simulink model "State_Machine_Harness_Dashboard"  (R2019b)
settings: configuration reference "BMS_Sw_CodeGenConfig" (kept outside this file)
undefined symbols (not defined in the file): SRE
settings Model: DataDictionary=DD_State_Machine.sldd  Creator=falderis  LastModifiedBy=cpatel
settings ConfigSetRef: SourceName=BMS_Sw_CodeGenConfig

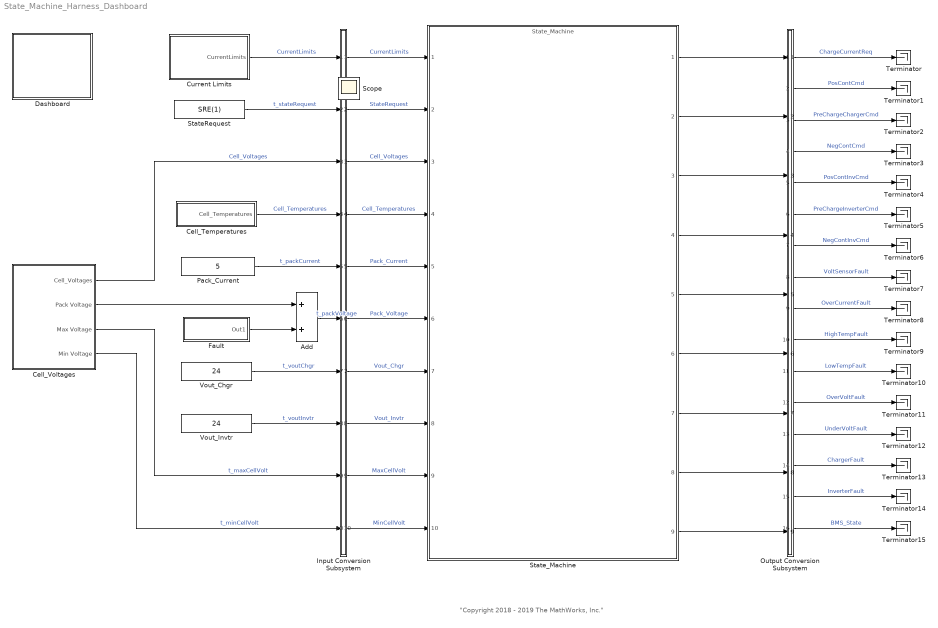
== system State_Machine_Harness_Dashboard ==
  note: "Copyright 2018 - 2019 The MathWorks, Inc."
  Add : Sum
  Cell_Temperatures : Subsystem
  Cell_Voltages : Subsystem
  Current Limits : Subsystem
  Dashboard : Subsystem
  Fault : Subsystem
  Input Conversion Subsystem : Subsystem  Tag=__SLT_ICS__  Description=|
      | Signal spec.
      | and routing
      settings: AttributesFormatString=%<Description>
  Output Conversion Subsystem : Subsystem  Tag=__SLT_OCS__  Description=|
      | Signal spec.
      | and routing
      settings: AttributesFormatString=%<Description>
  Pack_Current : Constant  Value=5  OutDataTypeStr=single  SampleTime=0.1
  StateRequest : Constant  Value=SRE(1)  OutDataTypeStr=Enum: SRE  SampleTime=0.1
  State_Machine : ModelReference  ModelNameDialog=State_Machine  SimulationMode=Normal  ModelReferenceVersion=1.640
  Terminator{,1..15} (16 alike) : Terminator
  Vout_Chgr : Constant  Value=24  OutDataTypeStr=single  SampleTime=0.1
  Vout_Invtr : Constant  Value=24  OutDataTypeStr=single  SampleTime=0.1
  Scope : Scope
  wires:
  Output Conversion Subsystem/1(Outport_1) -> Terminator/1  "ChargeCurrentReq"
  Output Conversion Subsystem/2(Outport_2) -> Terminator1/1  "PosContCmd"
  Output Conversion Subsystem/3(Outport_3) -> Terminator2/1  "PreChargeChargerCmd"
  Output Conversion Subsystem/4(Outport_4) -> Terminator3/1  "NegContCmd"
  Output Conversion Subsystem/5(Outport_5) -> Terminator4/1  "PosContInvCmd"
  Output Conversion Subsystem/6(Outport_6) -> Terminator5/1  "PreChargeInverterCmd"
  Output Conversion Subsystem/7(Outport_7) -> Terminator6/1  "NegContInvCmd"
  Output Conversion Subsystem/8(Outport_8) -> Terminator7/1  "VoltSensorFault"
  Output Conversion Subsystem/9(Outport_9) -> Terminator8/1  "OverCurrentFault"
  Output Conversion Subsystem/10(Outport_10) -> Terminator9/1  "HighTempFault"
  Output Conversion Subsystem/11(Outport_11) -> Terminator10/1  "LowTempFault"
  Output Conversion Subsystem/12(Outport_12) -> Terminator11/1  "OverVoltFault"
  Output Conversion Subsystem/13(Outport_13) -> Terminator12/1  "UnderVoltFault"
  Output Conversion Subsystem/14(Outport_14) -> Terminator13/1  "ChargerFault"
  Output Conversion Subsystem/15(Outport_15) -> Terminator14/1  "InverterFault"
  Output Conversion Subsystem/16(Outport_16) -> Terminator15/1  "BMS_State"
  Input Conversion Subsystem/1(Outport_1) -> State_Machine/1  "CurrentLimits"
  Input Conversion Subsystem/2(Outport_2) -> State_Machine/2  "StateRequest"
  Input Conversion Subsystem/3(Outport_3) -> State_Machine/3  "Cell_Voltages"
  Input Conversion Subsystem/4(Outport_4) -> State_Machine/4  "Cell_Temperatures"
  Input Conversion Subsystem/5(Outport_5) -> State_Machine/5  "Pack_Current"
  Input Conversion Subsystem/6(Outport_6) -> State_Machine/6  "Pack_Voltage"
  Input Conversion Subsystem/7(Outport_7) -> State_Machine/7  "Vout_Chgr"
  Input Conversion Subsystem/8(Outport_8) -> State_Machine/8  "Vout_Invtr"
  Input Conversion Subsystem/9(Outport_9) -> State_Machine/9  "MaxCellVolt"
  Input Conversion Subsystem/10(Outport_10) -> State_Machine/10  "MinCellVolt"
  State_Machine/1 -> Output Conversion Subsystem/1(Inport_1)
  State_Machine/2 -> Output Conversion Subsystem/2(Inport_2)
  State_Machine/3 -> Output Conversion Subsystem/3(Inport_3)
  State_Machine/4 -> Output Conversion Subsystem/4(Inport_4)
  State_Machine/5 -> Output Conversion Subsystem/5(Inport_5)
  State_Machine/6 -> Output Conversion Subsystem/6(Inport_6)
  State_Machine/7 -> Output Conversion Subsystem/7(Inport_7)
  State_Machine/8 -> Output Conversion Subsystem/8(Inport_8)
  State_Machine/9 -> Output Conversion Subsystem/9(Inport_9)
  Cell_Voltages/3(Max Voltage) -> Input Conversion Subsystem/9(Inport_9)  "t_maxCellVolt"
  Vout_Invtr/1 -> Input Conversion Subsystem/8(Inport_8)  "t_voutInvtr"
  Vout_Chgr/1 -> Input Conversion Subsystem/7(Inport_7)  "t_voutChgr"
  StateRequest/1 -> Input Conversion Subsystem/2(Inport_2)  "t_stateRequest"
  Cell_Voltages/4(Min Voltage) -> Input Conversion Subsystem/10(Inport_10)  "t_minCellVolt"
  Add/1 -> Input Conversion Subsystem/6(Inport_6)  "t_packVoltage"
  Current Limits/1(CurrentLimits) -> Input Conversion Subsystem/1(Inport_1)  "CurrentLimits"
  Cell_Temperatures/1(Cell_Temperatures) -> Input Conversion Subsystem/4(Inport_4)  "Cell_Temperatures"
  Cell_Voltages/1(Cell_Voltages) -> Input Conversion Subsystem/3(Inport_3)  "Cell_Voltages"
  Pack_Current/1 -> Input Conversion Subsystem/5(Inport_5)  "t_packCurrent"
  Cell_Voltages/2(Pack Voltage) -> Add/1
  Fault/1(Out1) -> Add/2

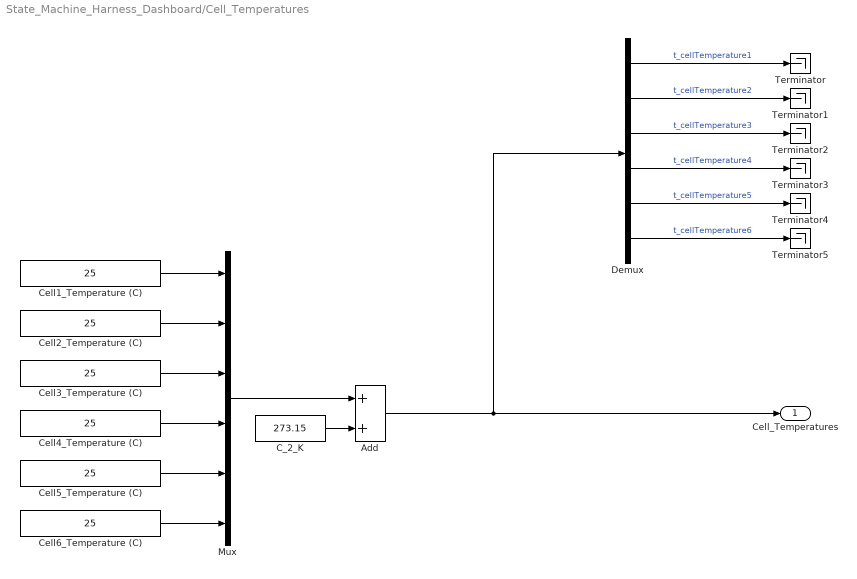
== system State_Machine_Harness_Dashboard/Cell_Temperatures ==
  Add : Sum
  C_2_K : Constant  Value=273.15  OutDataTypeStr=single  SampleTime=0.1
  Cell1_Temperature (C) : Constant  Value=25  OutDataTypeStr=single  SampleTime=0.1
  Cell2_Temperature (C) : Constant  Value=25  OutDataTypeStr=single  SampleTime=0.1
  Cell3_Temperature (C) : Constant  Value=25  OutDataTypeStr=single  SampleTime=0.1
  Cell4_Temperature (C) : Constant  Value=25  OutDataTypeStr=single  SampleTime=0.1
  Cell5_Temperature (C) : Constant  Value=25  OutDataTypeStr=single  SampleTime=0.1
  Cell6_Temperature (C) : Constant  Value=25  OutDataTypeStr=single  SampleTime=0.1
  Demux : Demux  Outputs=6
  Mux : Mux  Inputs=6
  Terminator{,1..5} (6 alike) : Terminator
  Cell_Temperatures : Outport  VectorParamsAs1DForOutWhenUnconnected=off
  wires:
  Add/1 -> Demux/1, Cell_Temperatures/1
  Cell3_Temperature (C)/1 -> Mux/3
  C_2_K/1 -> Add/2
  Cell2_Temperature (C)/1 -> Mux/2
  Cell4_Temperature (C)/1 -> Mux/4
  Cell5_Temperature (C)/1 -> Mux/5
  Mux/1 -> Add/1
  Cell6_Temperature (C)/1 -> Mux/6
  Cell1_Temperature (C)/1 -> Mux/1
  Demux/1 -> Terminator/1  "t_cellTemperature1"
  Demux/2 -> Terminator1/1  "t_cellTemperature2"
  Demux/3 -> Terminator2/1  "t_cellTemperature3"
  Demux/4 -> Terminator3/1  "t_cellTemperature4"
  Demux/5 -> Terminator4/1  "t_cellTemperature5"
  Demux/6 -> Terminator5/1  "t_cellTemperature6"

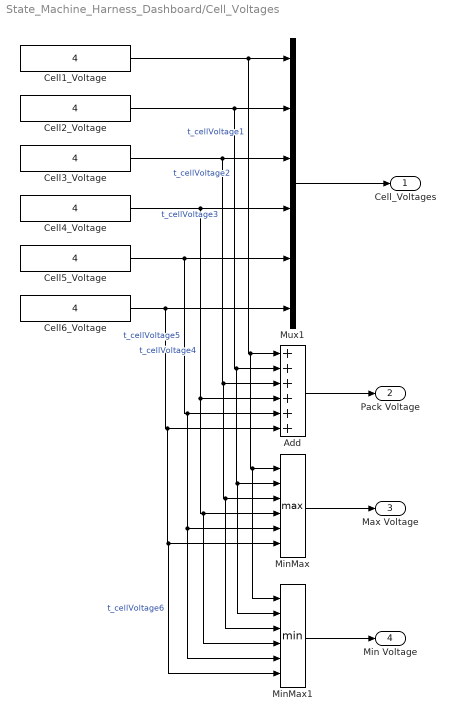
== system State_Machine_Harness_Dashboard/Cell_Voltages ==
  Add : Sum  Inputs=6
  Cell1_Voltage : Constant  Value=4  OutDataTypeStr=single  SampleTime=0.1
  Cell2_Voltage : Constant  Value=4  OutDataTypeStr=single  SampleTime=0.1
  Cell3_Voltage : Constant  Value=4  OutDataTypeStr=single  SampleTime=0.1
  Cell4_Voltage : Constant  Value=4  OutDataTypeStr=single  SampleTime=0.1
  Cell5_Voltage : Constant  Value=4  OutDataTypeStr=single  SampleTime=0.1
  Cell6_Voltage : Constant  Value=4  OutDataTypeStr=single  SampleTime=0.1
  MinMax : MinMax  Function=max  Inputs=6
  MinMax1 : MinMax  Inputs=6
  Mux1 : Mux  Inputs=6
  Cell_Voltages : Outport  VectorParamsAs1DForOutWhenUnconnected=off
  Pack Voltage : Outport  Port=2  VectorParamsAs1DForOutWhenUnconnected=off
  Max Voltage : Outport  Port=3  VectorParamsAs1DForOutWhenUnconnected=off
  Min Voltage : Outport  Port=4  VectorParamsAs1DForOutWhenUnconnected=off
  wires:
  Cell6_Voltage/1 -> MinMax1/6, MinMax/6, Add/6, Mux1/6  "t_cellVoltage6"
  Cell3_Voltage/1 -> MinMax1/3, MinMax/3, Add/3, Mux1/3  "t_cellVoltage3"
  Cell2_Voltage/1 -> MinMax1/2, MinMax/2, Add/2, Mux1/2  "t_cellVoltage2"
  Mux1/1 -> Cell_Voltages/1
  Cell1_Voltage/1 -> MinMax1/1, MinMax/1, Add/1, Mux1/1  "t_cellVoltage1"
  Cell5_Voltage/1 -> MinMax1/5, MinMax/5, Add/5, Mux1/5  "t_cellVoltage5"
  Cell4_Voltage/1 -> MinMax1/4, MinMax/4, Add/4, Mux1/4  "t_cellVoltage4"
  Add/1 -> Pack Voltage/1
  MinMax/1 -> Max Voltage/1
  MinMax1/1 -> Min Voltage/1

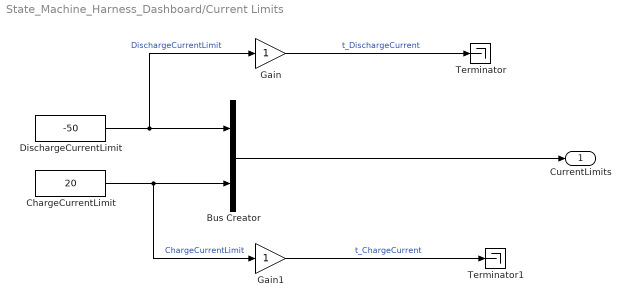
== system State_Machine_Harness_Dashboard/Current Limits ==
  Bus Creator : BusCreator  Inputs=2  OutDataTypeStr=Bus: CurrentLimits
  ChargeCurrentLimit : Constant  Value=20  OutDataTypeStr=single  SampleTime=0.1
  DischargeCurrentLimit : Constant  Value=-50  OutDataTypeStr=single  SampleTime=0.1
  Gain : Gain
  Gain1 : Gain
  Terminator : Terminator
  Terminator1 : Terminator
  CurrentLimits : Outport  VectorParamsAs1DForOutWhenUnconnected=off
  wires:
  Bus Creator/1 -> CurrentLimits/1
  DischargeCurrentLimit/1 -> Gain/1, Bus Creator/1  "DischargeCurrentLimit"
  ChargeCurrentLimit/1 -> Gain1/1, Bus Creator/2  "ChargeCurrentLimit"
  Gain/1 -> Terminator/1  "t_DischargeCurrent"
  Gain1/1 -> Terminator1/1  "t_ChargeCurrent"

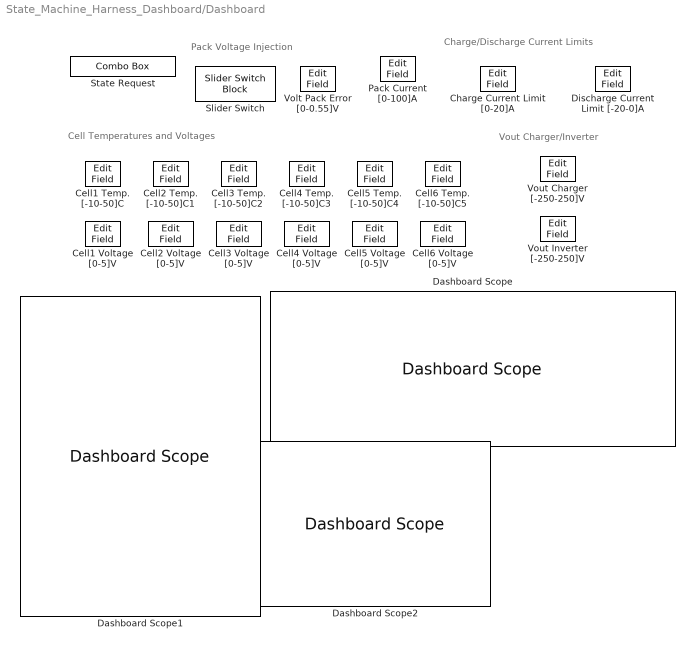
== system State_Machine_Harness_Dashboard/Dashboard ==
  note: Pack Voltage Injection
  note: Cell Temperatures and Voltages
  note: Vout Charger/Inverter
  note: Charge/Discharge Current Limits
  Cell1 Temp. [-10-50]C : EditField  LabelPosition=Hide  ShowInitialText=on  Alignment=Center
  Cell1 Voltage [0-5]V : EditField  LabelPosition=Hide  ShowInitialText=on  Alignment=Center
  Cell2 Temp. [-10-50]C1 : EditField  LabelPosition=Hide  ShowInitialText=on  Alignment=Center
  Cell2 Voltage [0-5]V : EditField  LabelPosition=Hide  ShowInitialText=on  Alignment=Center
  Cell3 Temp. [-10-50]C2 : EditField  LabelPosition=Hide  ShowInitialText=on  Alignment=Center
  Cell3 Voltage [0-5]V : EditField  LabelPosition=Hide  ShowInitialText=on  Alignment=Center
  Cell4 Temp. [-10-50]C3 : EditField  LabelPosition=Hide  ShowInitialText=on  Alignment=Center
  Cell4 Voltage [0-5]V : EditField  LabelPosition=Hide  ShowInitialText=on  Alignment=Center
  Cell5 Temp. [-10-50]C4 : EditField  LabelPosition=Hide  ShowInitialText=on  Alignment=Center
  Cell5 Voltage [0-5]V : EditField  LabelPosition=Hide  ShowInitialText=on  Alignment=Center
  Cell6 Temp. [-10-50]C5 : EditField  LabelPosition=Hide  ShowInitialText=on  Alignment=Center
  Cell6 Voltage [0-5]V : EditField  LabelPosition=Hide  ShowInitialText=on  Alignment=Center
  Charge Current Limit [0-20]A : EditField  LabelPosition=Hide  ShowInitialText=on  Alignment=Center
  Dashboard Scope : DashboardScope  TimeSpan=50  ScaleAtStop=off
  Dashboard Scope1 : DashboardScope  TimeSpan=50  Ymin=0  Ymax=1.2
  Dashboard Scope2 : DashboardScope  TimeSpan=50  Ymin=0  Ymax=35
  Discharge Current Limit [-20-0]A : EditField  LabelPosition=Hide  ShowInitialText=on  Alignment=Center
  Pack Current [0-100]A : EditField  LabelPosition=Hide  ShowInitialText=on  Alignment=Center
  Slider Switch : SliderSwitchBlock
      settings: Values={{'Off', 'On'}, [0 1]}
  State Request : ComboBox  LabelPosition=Hide  SelectedLabel=Charging
      settings: Values={{'Balancing', 'Charging', 'Driving'}, [0 1 2]}
  Volt Pack Error [0-0.55]V : EditField  LabelPosition=Hide  ShowInitialText=on  Alignment=Center
  Vout Charger [-250-250]V : EditField  LabelPosition=Hide  ShowInitialText=on  Alignment=Center
  Vout Inverter [-250-250]V : EditField  LabelPosition=Hide  ShowInitialText=on  Alignment=Center

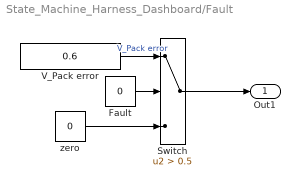
== system State_Machine_Harness_Dashboard/Fault ==
  Fault : Constant  Value=0  OutDataTypeStr=boolean  LockScale=on
  Switch : Switch  Criteria=u2 > Threshold  Threshold=0.5
  V_Pack error : Constant  Value=0.6  OutDataTypeStr=single  SampleTime=0.1
  zero : Constant  Value=0  OutDataTypeStr=single  LockScale=on
  Out1 : Outport  VectorParamsAs1DForOutWhenUnconnected=off
  wires:
  V_Pack error/1 -> Switch/1  "V_Pack error"
  zero/1 -> Switch/3
  Fault/1 -> Switch/2
  Switch/1 -> Out1/1

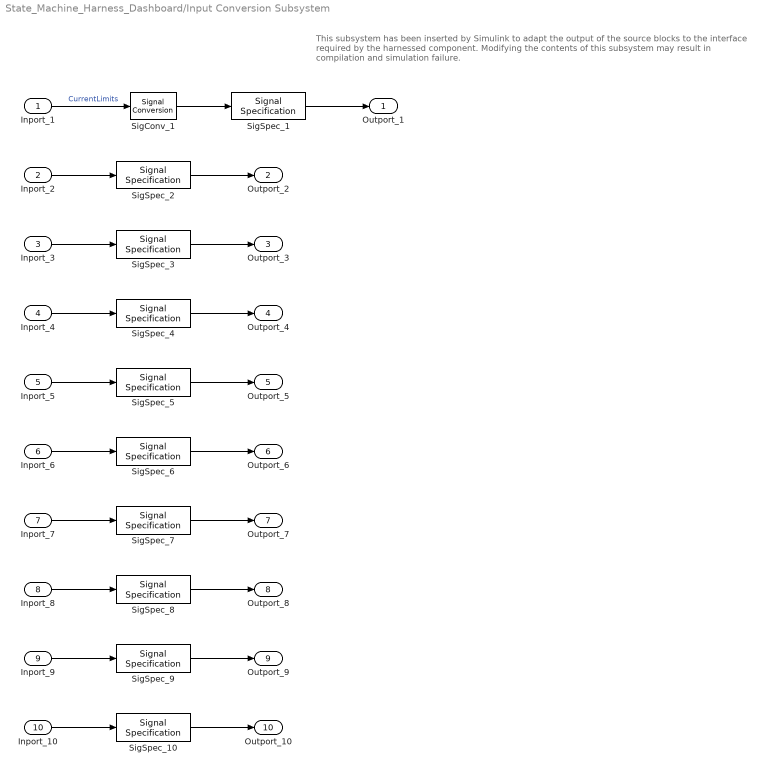
== system State_Machine_Harness_Dashboard/Input Conversion Subsystem ==
  note: This subsystem has been inserted by Simulink to adapt the output of the source blocks to the interface required by the harnessed component.
      |  Modifying the contents of this subsystem may result in compilation and simulation failure.
  Inport_1 : Inport
  Inport_2 : Inport  Port=2
  Inport_3 : Inport  Port=3
  Inport_4 : Inport  Port=4
  Inport_5 : Inport  Port=5
  Inport_6 : Inport  Port=6
  Inport_7 : Inport  Port=7
  Inport_8 : Inport  Port=8
  Inport_9 : Inport  Port=9
  Inport_10 : Inport  Port=10
  SigConv_1 : SignalConversion  ConversionOutput=Virtual bus  OverrideOpt=off
  SigSpec_1 : SignalSpecification  OutDataTypeStr=Bus: CurrentLimits  SampleTime=0.1
  SigSpec_{5..10} (6 alike) : SignalSpecification  OutDataTypeStr=single  Dimensions=[1]  SampleTime=0.1
  SigSpec_2 : SignalSpecification  OutDataTypeStr=Enum: SRE  Dimensions=[1]  SampleTime=0.1
  SigSpec_3 : SignalSpecification  OutDataTypeStr=single  Dimensions=[6]  SampleTime=0.1
  SigSpec_4 : SignalSpecification  OutDataTypeStr=single  Dimensions=[6]  SampleTime=0.1
  Outport_1 : Outport  VectorParamsAs1DForOutWhenUnconnected=off
  Outport_2 : Outport  Port=2  VectorParamsAs1DForOutWhenUnconnected=off
  Outport_3 : Outport  Port=3  VectorParamsAs1DForOutWhenUnconnected=off
  Outport_4 : Outport  Port=4  VectorParamsAs1DForOutWhenUnconnected=off
  Outport_5 : Outport  Port=5  VectorParamsAs1DForOutWhenUnconnected=off
  Outport_6 : Outport  Port=6  VectorParamsAs1DForOutWhenUnconnected=off
  Outport_7 : Outport  Port=7  VectorParamsAs1DForOutWhenUnconnected=off
  Outport_8 : Outport  Port=8  VectorParamsAs1DForOutWhenUnconnected=off
  Outport_9 : Outport  Port=9  VectorParamsAs1DForOutWhenUnconnected=off
  Outport_10 : Outport  Port=10  VectorParamsAs1DForOutWhenUnconnected=off
  wires:
  SigSpec_1/1 -> Outport_1/1
  SigConv_1/1 -> SigSpec_1/1
  Inport_1/1 -> SigConv_1/1  "CurrentLimits"
  SigSpec_2/1 -> Outport_2/1
  Inport_2/1 -> SigSpec_2/1
  SigSpec_3/1 -> Outport_3/1
  Inport_3/1 -> SigSpec_3/1
  SigSpec_4/1 -> Outport_4/1
  Inport_4/1 -> SigSpec_4/1
  SigSpec_5/1 -> Outport_5/1
  Inport_5/1 -> SigSpec_5/1
  SigSpec_6/1 -> Outport_6/1
  Inport_6/1 -> SigSpec_6/1
  SigSpec_7/1 -> Outport_7/1
  Inport_7/1 -> SigSpec_7/1
  SigSpec_8/1 -> Outport_8/1
  Inport_8/1 -> SigSpec_8/1
  SigSpec_9/1 -> Outport_9/1
  Inport_9/1 -> SigSpec_9/1
  SigSpec_10/1 -> Outport_10/1
  Inport_10/1 -> SigSpec_10/1

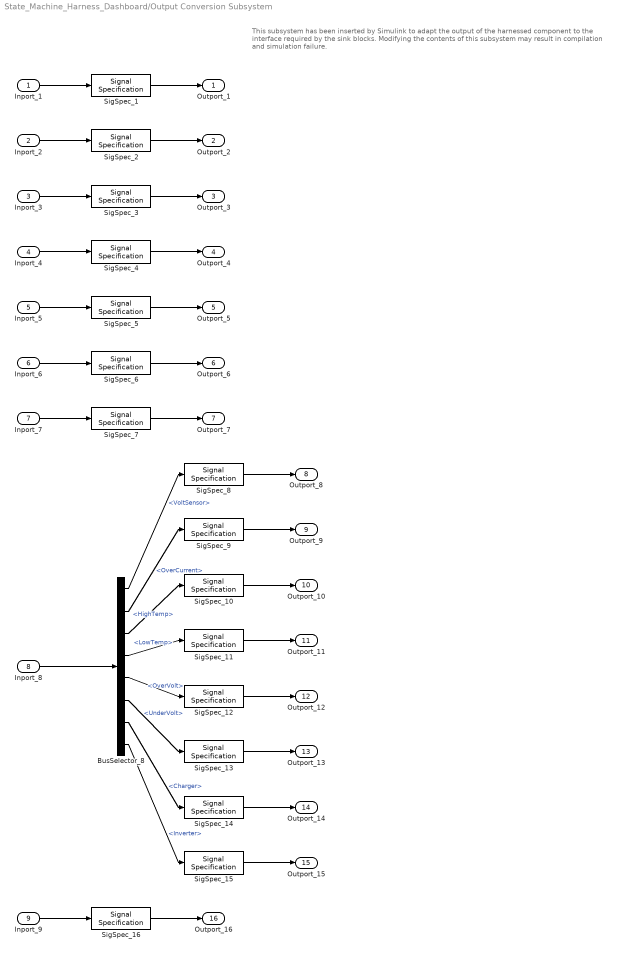
== system State_Machine_Harness_Dashboard/Output Conversion Subsystem ==
  note: This subsystem has been inserted by Simulink to adapt the output of the harnessed component to the interface required by the sink blocks.
      |  Modifying the contents of this subsystem may result in compilation and simulation failure.
  Inport_1 : Inport
  Inport_2 : Inport  Port=2
  Inport_3 : Inport  Port=3
  Inport_4 : Inport  Port=4
  Inport_5 : Inport  Port=5
  Inport_6 : Inport  Port=6
  Inport_7 : Inport  Port=7
  Inport_8 : Inport  Port=8
  Inport_9 : Inport  Port=9
  BusSelector_8 : BusSelector  OutputSignals=VoltSensor,OverCurrent,HighTemp,LowTemp,OverVolt,UnderVolt,Charger,Inverter
  SigSpec_1 : SignalSpecification  OutDataTypeStr=single  Dimensions=[1]  SampleTime=0.1
  SigSpec_{2..15} (14 alike) : SignalSpecification  OutDataTypeStr=boolean  Dimensions=[1]  SampleTime=0.1
  SigSpec_16 : SignalSpecification  OutDataTypeStr=Enum: BMS_State_Enum  Dimensions=[1]  SampleTime=0.1
  Outport_1 : Outport  VectorParamsAs1DForOutWhenUnconnected=off
  Outport_2 : Outport  Port=2  VectorParamsAs1DForOutWhenUnconnected=off
  Outport_3 : Outport  Port=3  VectorParamsAs1DForOutWhenUnconnected=off
  Outport_4 : Outport  Port=4  VectorParamsAs1DForOutWhenUnconnected=off
  Outport_5 : Outport  Port=5  VectorParamsAs1DForOutWhenUnconnected=off
  Outport_6 : Outport  Port=6  VectorParamsAs1DForOutWhenUnconnected=off
  Outport_7 : Outport  Port=7  VectorParamsAs1DForOutWhenUnconnected=off
  Outport_8 : Outport  Port=8  VectorParamsAs1DForOutWhenUnconnected=off
  Outport_9 : Outport  Port=9  VectorParamsAs1DForOutWhenUnconnected=off
  Outport_10 : Outport  Port=10  VectorParamsAs1DForOutWhenUnconnected=off
  Outport_11 : Outport  Port=11  VectorParamsAs1DForOutWhenUnconnected=off
  Outport_12 : Outport  Port=12  VectorParamsAs1DForOutWhenUnconnected=off
  Outport_13 : Outport  Port=13  VectorParamsAs1DForOutWhenUnconnected=off
  Outport_14 : Outport  Port=14  VectorParamsAs1DForOutWhenUnconnected=off
  Outport_15 : Outport  Port=15  VectorParamsAs1DForOutWhenUnconnected=off
  Outport_16 : Outport  Port=16  VectorParamsAs1DForOutWhenUnconnected=off
  wires:
  Inport_1/1 -> SigSpec_1/1
  SigSpec_1/1 -> Outport_1/1
  Inport_2/1 -> SigSpec_2/1
  SigSpec_2/1 -> Outport_2/1
  Inport_3/1 -> SigSpec_3/1
  SigSpec_3/1 -> Outport_3/1
  Inport_4/1 -> SigSpec_4/1
  SigSpec_4/1 -> Outport_4/1
  Inport_5/1 -> SigSpec_5/1
  SigSpec_5/1 -> Outport_5/1
  Inport_6/1 -> SigSpec_6/1
  SigSpec_6/1 -> Outport_6/1
  Inport_7/1 -> SigSpec_7/1
  SigSpec_7/1 -> Outport_7/1
  Inport_8/1 -> BusSelector_8/1
  BusSelector_8/1 -> SigSpec_8/1  "<VoltSensor>"
  SigSpec_8/1 -> Outport_8/1
  BusSelector_8/2 -> SigSpec_9/1  "<OverCurrent>"
  SigSpec_9/1 -> Outport_9/1
  BusSelector_8/3 -> SigSpec_10/1  "<HighTemp>"
  SigSpec_10/1 -> Outport_10/1
  BusSelector_8/4 -> SigSpec_11/1  "<LowTemp>"
  SigSpec_11/1 -> Outport_11/1
  BusSelector_8/5 -> SigSpec_12/1  "<OverVolt>"
  SigSpec_12/1 -> Outport_12/1
  BusSelector_8/6 -> SigSpec_13/1  "<UnderVolt>"
  SigSpec_13/1 -> Outport_13/1
  BusSelector_8/7 -> SigSpec_14/1  "<Charger>"
  SigSpec_14/1 -> Outport_14/1
  BusSelector_8/8 -> SigSpec_15/1  "<Inverter>"
  SigSpec_15/1 -> Outport_15/1
  Inport_9/1 -> SigSpec_16/1
  SigSpec_16/1 -> Outport_16/1
